simulink model "complete_plant_ediff_conflict_copy_Ethan’s MacBook Pro_2022_11_12"  (R2022b)
settings: Solver=FixedStepAuto  StartTime=0.0  StopTime=300  RelTol=1e-3  EnableMultiTasking=on
model workspace (MAT data in the model file):
  A = 1.0221
  A1 = Simulink.Parameter
  A1.Value = 39.8344
  A1.DataType = 'auto'
  A1.Complexity = 'real'
  A1.Dimensions = [1 1]
  A2 = Simulink.Parameter
  A2.Value = 813.078
  A2.DataType = 'auto'
  A2.Complexity = 'real'
  A2.Dimensions = [1 1]
  ALL_TRACK_DATA.track_data_Left = [Inf Inf Inf Inf Inf Inf Inf Inf Inf Inf Inf Inf ... (182152 elements, 22769x8)]
  ALL_TRACK_DATA.track_data_Right = [Inf Inf Inf Inf Inf Inf Inf Inf Inf Inf Inf Inf ... (182152 elements, 22769x8)]
  ALL_TRACK_DATA.track_data_acceleration = [Inf Inf Inf Inf Inf Inf Inf Inf Inf Inf Inf Inf ... (6008 elements, 751x8)]
  ALL_TRACK_DATA.track_data_endurance = [Inf -1348.33962917 -674.16944376 -449.445883811 -337.083980227 -269.666739189 -224.721829424 -192.618251815 -168.540506804 -149.813316856 -134.831515454 -122.573632994 ... (77796 elements, 19449x4)]
  ALL_TRACK_DATA.track_data_grand_prix = [Inf Inf Inf Inf Inf Inf Inf Inf Inf Inf Inf Inf ... (33752 elements, 4219x8)]
  ALL_TRACK_DATA.track_data_skidpad = [Inf Inf Inf Inf Inf Inf Inf Inf Inf Inf Inf Inf ... (18312 elements, 2289x8)]
  Af = 1.0221
  B1 = Simulink.Parameter
  B1.Value = 1.287e-06
  B1.DataType = 'auto'
  B1.Complexity = 'real'
  B1.Dimensions = [1 1]
  B2 = Simulink.Parameter
  B2.Value = -0.002325
  B2.DataType = 'auto'
  B2.Complexity = 'real'
  B2.Dimensions = [1 1]
  B3 = Simulink.Parameter
  B3.Value = 3.797
  B3.DataType = 'auto'
  B3.Complexity = 'real'
  B3.Dimensions = [1 1]
  BattCap = 16
  BattCap_I = 16
  C1 = Simulink.Parameter
  C1.Value = -2.541e-09
  C1.DataType = 'auto'
  C1.Complexity = 'real'
  C1.Dimensions = [1 1]
  C2 = Simulink.Parameter
  C2.Value = 5.279e-06
  C2.DataType = 'auto'
  C2.Complexity = 'real'
  C2.Dimensions = [1 1]
  C3 = Simulink.Parameter
  C3.Value = -0.003943
  C3.DataType = 'auto'
  C3.Complexity = 'real'
  C3.Dimensions = [1 1]
  C4 = Simulink.Parameter
  C4.Value = 3.634
  C4.DataType = 'auto'
  C4.Complexity = 'real'
  C4.Dimensions = [1 1]
  C_param = Simulink.Parameter
  C_param.Value = [0 13757.41 21278.97 26666.02 30253.47 30313.18 30313.18]
  C_param.DataType = 'auto'
  C_param.Complexity = 'real'
  C_param.Dimensions = [1 7]
  Cd = 1.149
  FZ_C = Simulink.Parameter
  FZ_C.Value = [0 204.13 427.04 668.1 895.72 1124.4 1324.4]
  FZ_C.DataType = 'auto'
  FZ_C.Complexity = 'real'
  FZ_C.Dimensions = [1 7]
  Fx_limit = Simulink.Parameter
  Fx_limit.Value = [300 300]
  Fx_limit.DataType = 'auto'
  Fx_limit.Complexity = 'real'
  Fx_limit.Dimensions = [1 2]
  I = Simulink.Parameter
  I.Value = 60
  I.DataType = 'auto'
  I.Complexity = 'real'
  I.Dimensions = [1 1]
  IYY_Tire = 0.3
  J_z = Simulink.Parameter
  J_z.Value = 75
  J_z.DataType = 'auto'
  J_z.Complexity = 'real'
  J_z.Dimensions = [1 1]
  Ku = Simulink.Parameter
  Ku.Value = 0.0509683995923
  Ku.DataType = 'auto'
  Ku.Complexity = 'real'
  Ku.Dimensions = [1 1]
  Motor_T_I = [30 30]
  Np = 4
  Ns = 80
  P = Simulink.Parameter
  P.Value = 3
  P.DataType = 'auto'
  P.Complexity = 'real'
  P.Dimensions = [1 1]
  RE = Simulink.Parameter
  RE.Value = 0.2228169203
  RE.DataType = 'auto'
  RE.Complexity = 'real'
  RE.Dimensions = [1 1]
  RIM_RADIUS = 0.1524
  Rm = 0.079375
  S1 = Simulink.Parameter
  S1.Value = 7e-05
  S1.DataType = 'auto'
  S1.Complexity = 'real'
  S1.Dimensions = [1 1]
  S2 = Simulink.Parameter
  S2.Value = -0.0038
  S2.DataType = 'auto'
  S2.Complexity = 'real'
  S2.Dimensions = [1 1]
  S3 = Simulink.Parameter
  S3.Value = 0.6535
  S3.DataType = 'auto'
  S3.Complexity = 'real'
  S3.Dimensions = [1 1]
  S4 = Simulink.Parameter
  S4.Value = 0.1061
  S4.DataType = 'auto'
  S4.Complexity = 'real'
  S4.Dimensions = [1 1]
  SL_limit = Simulink.Parameter
  SL_limit.Value = 0.3
  SL_limit.DataType = 'auto'
  SL_limit.Complexity = 'real'
  SL_limit.Dimensions = [1 1]
  T = Simulink.Parameter
  T.Value = 0
  T.DataType = 'single'
  T.Complexity = 'real'
  T.Dimensions = [1 1]
  T2F = Simulink.Parameter
  T2F.Value = [4.38500022888 4.38500022888 4.38500022888 4.38500022888]
  T2F.DataType = 'single'
  T2F.Complexity = 'real'
  T2F.Dimensions = [1 4]
  Tair = 293
  V_target = Simulink.Parameter
  V_target.Value = [0 3 6 9 12 15 18 21 25 31]
  V_target.DataType = 'auto'
  V_target.Complexity = 'real'
  V_target.Dimensions = [1 10]
  Vg_ref = 10
  Vth = Simulink.Parameter
  Vth.Value = 2
  Vth.DataType = 'auto'
  Vth.Complexity = 'real'
  Vth.Dimensions = [1 1]
  Vx_I = 0
  Vy_I = 0
  WHEEL_WIDTH = 0.1524
  a = Simulink.Parameter
  a.Value = 1.14
  a.DataType = 'auto'
  a.Complexity = 'real'
  a.Dimensions = [1 1]
  abs_max_torque = Simulink.Parameter
  abs_max_torque.Value = [25 25 25 25]
  abs_max_torque.DataType = 'auto'
  abs_max_torque.Complexity = 'real'
  abs_max_torque.Dimensions = [1 4]
  absolute_battery_power_limits = Simulink.Parameter
  absolute_battery_power_limits.Value = [75000 -700]
  absolute_battery_power_limits.DataType = 'auto'
  absolute_battery_power_limits.Complexity = 'real'
  absolute_battery_power_limits.Dimensions = [1 2]
  b = Simulink.Parameter
  b.Value = -0.03291
  b.DataType = 'auto'
  b.Complexity = 'real'
  b.Dimensions = [1 1]
  brake_bias = [0.65 0.65 0.35 0.35]
  brakecoeff = Simulink.Parameter
  brakecoeff.Value = [61.33 61.33 40.54 40.54]
  brakecoeff.DataType = 'auto'
  brakecoeff.Complexity = 'real'
  brakecoeff.Dimensions = [1 4]
  c = Simulink.Parameter
  c.Value = -1.14
  c.DataType = 'auto'
  c.Complexity = 'real'
  c.Dimensions = [1 1]
  cl = 2.11014
  d = Simulink.Parameter
  d.Value = -1.027
  d.DataType = 'auto'
  d.Complexity = 'real'
  d.Dimensions = [1 1]
  dTx = Simulink.Parameter
  dTx.Value = 0.01
  dTx.DataType = 'auto'
  dTx.Complexity = 'real'
  dTx.Dimensions = [1 1]
  dZ = 0.295
  d_bore = 0.0254
  deadband_angle = Simulink.Parameter
  deadband_angle.Value = 4
  deadband_angle.DataType = 'auto'
  deadband_angle.Complexity = 'real'
  deadband_angle.Dimensions = [1 1]
  deadband_velocity = Simulink.Parameter
  deadband_velocity.Value = 0.5
  deadband_velocity.DataType = 'auto'
  deadband_velocity.Complexity = 'real'
  deadband_velocity.Dimensions = [1 1]
  deg2rad = Simulink.Parameter
  deg2rad.Value = 0.01745329
  deg2rad.DataType = 'auto'
  deg2rad.Complexity = 'real'
  deg2rad.Dimensions = [1 1]
  di2bp = 20
  distance_traveled = 75
  efficiency_grid = Simulink.Parameter
  efficiency_grid.Value = [0.011 0.0107113163972 0.0104226327945 0.0101339491917 0.01 0.01 0.01 0.01 0.01 0.01 0.01 0.01 ... (26857 elements, 107x251)]
  efficiency_grid.DataType = 'auto'
  efficiency_grid.Complexity = 'real'
  efficiency_grid.Dimensions = [107 251]
  g = Simulink.Parameter
  g.Value = 9.81
  g.DataType = 'auto'
  g.Complexity = 'real'
  g.Dimensions = [1 1]
  gr = Simulink.Parameter
  gr.Value = [6.63043 6.63043 8 8]
  gr.DataType = 'auto'
  gr.Complexity = 'real'
  gr.Dimensions = [1 4]
  inch2mm = Simulink.Parameter
  inch2mm.Value = 25.4
  inch2mm.DataType = 'auto'
  inch2mm.Complexity = 'real'
  inch2mm.Dimensions = [1 1]
  k_limit = Simulink.Parameter
  k_limit.Value = 3.461
  k_limit.DataType = 'auto'
  k_limit.Complexity = 'real'
  k_limit.Dimensions = [1 1]
  kx = 200
  l = Simulink.Parameter
  l.Value = [0.7922471 0.7828529]
  l.DataType = 'auto'
  l.Complexity = 'real'
  l.Dimensions = [1 2]
  lateral_coeff = Simulink.Parameter
  lateral_coeff.Value = 1
  lateral_coeff.DataType = 'auto'
  lateral_coeff.Complexity = 'real'
  lateral_coeff.Dimensions = [1 1]
  m = 320
  m_tire_f = 6
  m_tire_r = 16
  max_delta_omega = Simulink.Parameter
  max_delta_omega.Value = 5
  max_delta_omega.DataType = 'auto'
  max_delta_omega.Complexity = 'real'
  max_delta_omega.Dimensions = [1 1]
  max_motor_temp = Simulink.Parameter
  max_motor_temp.Value = 75
  max_motor_temp.DataType = 'auto'
  max_motor_temp.Complexity = 'real'
  max_motor_temp.Dimensions = [1 1]
  max_rpm = Simulink.Parameter
  max_rpm.Value = [0 841.626809471 843.653762207 845.894764963 848.156711672 850.460546282 852.795796818 855.162463281 857.571017646 860.010987937 862.492846131 865.016592226 867.582226224 870.189748124 872.839157925 875.530455629 878.274113209 881.070130668 883.908036029 886.798301266 889.740926382 892.735911375 895.793728221 898.903904944 902.076913521 905.302281975 908.590482282 911.941514442 915.355378455 918.832074321 922.37160204 925.984433588 929.670568964 933.419536193 937.252279226 941.147854111 945.116732826 949.169387344 953.295345691 957.494607867 961.777645846 970.595049217 975.129414609 979.747555804 984.449472804 989.245637583 994.125578166 999.099766529 1004.16820267 1009.33088659 1014.58781829 1019.93899777 1025.39489701 1030.94504402 1036.58943882 1042.34902534 1048.20285965 1054.16141371 1060.2351595 1066.41362504 1072.69681034 1079.09518737 1085.59828416 1092.21657267 1098.95005292 1105.80919687 1112.77306058 1138.42940056]
  max_rpm.DataType = 'auto'
  max_rpm.Complexity = 'real'
  max_rpm.Dimensions = [1 68]
  max_torque = Simulink.Parameter
  max_torque.Value = [25 25 24.669 24.305 23.939 23.571 23.202 22.83 22.458 22.084 21.708 21.331 20.953 20.574 20.194 19.813 19.431 19.048 18.665 18.281 17.897 17.512 17.127 16.742 16.356 15.971 15.586 15.2 14.815 14.431 14.047 13.663 13.28 12.897 12.516 12.135 11.755 11.376 10.999 10.622 10.247 9.501 9.131 8.762 8.395 8.029 7.666 7.305 6.946 6.589 6.234 5.882 5.532 5.185 4.84 4.499 4.16 3.824 3.491 3.161 2.834 2.511 2.191 1.875 1.562 1.252 0.947 0]
  max_torque.DataType = 'auto'
  max_torque.Complexity = 'real'
  max_torque.Dimensions = [1 68]
  max_yaw_field = Simulink.Parameter
  max_yaw_field.Value = [0.67 0.67 0.67 0.83 0.57 0.62 0.377 0.4245 0.425 0.425]
  max_yaw_field.DataType = 'auto'
  max_yaw_field.Complexity = 'real'
  max_yaw_field.Dimensions = [1 10]
  mcp_Motor = 573
  min_velocity_regen = Simulink.Parameter
  min_velocity_regen.Value = 1.4
  min_velocity_regen.DataType = 'auto'
  min_velocity_regen.Complexity = 'real'
  min_velocity_regen.Dimensions = [1 1]
  motor_efficiency = Simulink.Parameter
  motor_efficiency.Value = [0.95 0.95 0.95 0.95]
  motor_efficiency.DataType = 'auto'
  motor_efficiency.Complexity = 'real'
  motor_efficiency.Dimensions = [1 4]
  motor_enable = Simulink.Parameter
  motor_enable.Value = [0 0 1 1]
  motor_enable.DataType = 'auto'
  motor_enable.Complexity = 'real'
  motor_enable.Dimensions = [1 4]
  mu_factor = Simulink.Parameter
  mu_factor.Value = 0.7
  mu_factor.DataType = 'auto'
  mu_factor.Complexity = 'real'
  mu_factor.Dimensions = [1 1]
  mu_k_brake = 0.4
  mu_s_brake = 0.5
  power_input_grid = Simulink.Parameter
  power_input_grid.Value = [0 0 0 0 0 0 0 0 0 0 0 0 ... (26857 elements, 251x107)]
  power_input_grid.DataType = 'auto'
  power_input_grid.Complexity = 'real'
  power_input_grid.Dimensions = [251 107]
  power_loss_grid = Simulink.Parameter
  power_loss_grid.Value = [0.1 0.2 0.3 0.4 0.5 0.6 0.7 0.8 0.9 1 1.1 1.2 ... (26857 elements, 251x107)]
  power_loss_grid.DataType = 'auto'
  power_loss_grid.Complexity = 'real'
  power_loss_grid.Dimensions = [251 107]
  power_loss_limit = Simulink.Parameter
  power_loss_limit.Value = [0 0 5800 5800]
  power_loss_limit.DataType = 'auto'
  power_loss_limit.Complexity = 'real'
  power_loss_limit.Dimensions = [1 4]
  rho = 1.225
  rpm_index_calibration = Simulink.Parameter
  rpm_index_calibration.Value = 10.4719755
  rpm_index_calibration.DataType = 'auto'
  rpm_index_calibration.Complexity = 'real'
  rpm_index_calibration.Dimensions = [1 1]
  rpm_sweep = Simulink.Parameter
  rpm_sweep.Value = [0 10.4719755 20.943951 31.4159265 41.887902 52.3598775 62.831853 73.3038285 83.775804 94.2477795 104.719755 115.1917305 125.663706 136.1356815 146.607657 157.0796325 167.551608 178.0235835 188.495559 198.9675345 209.43951 219.9114855 230.383461 240.8554365 251.327412 261.7993875 272.271363 282.7433385 293.215314 303.6872895 314.159265 324.6312405 335.103216 345.5751915 356.047167 366.5191425 376.991118 387.4630935 397.935069 408.4070445 418.87902 429.3509955 439.822971 450.2949465 460.766922 471.2388975 481.710873 492.1828485 502.654824 513.1267995 523.598775 534.0707505 544.542726 555.0147015 565.486677 575.9586525 586.430628 596.9026035 607.374579 617.8465545 628.31853 638.7905055 649.262481 659.7344565 670.206432 680.6784075 691.150383 701.6223585 712.094334 722.5663095 733.038285 743.5102605 753.982236 764.4542115 774.926187 785.3981625 795.870138 806.3421135 816.814089 827.2860645 837.75804 848.2300155 858.701991 869.1739665 879.645942 890.1179175 900.589893 911.0618685 921.533844 932.0058195 942.477795 952.9497705 963.421746 973.8937215 984.365697 994.8376725 1005.309648 1015.7816235 1026.253599 1036.7255745 1047.19755 1057.6695255 1068.141501 1078.6134765 1089.085452 1099.5574275 1110.029403]
  rpm_sweep.DataType = 'auto'
  rpm_sweep.Complexity = 'real'
  rpm_sweep.Dimensions = [1 107]
  s = Simulink.Parameter
  s.Value = [0.647895 0.62102]
  s.DataType = 'auto'
  s.Complexity = 'real'
  s.Dimensions = [1 2]
  steer_slope = Simulink.Parameter
  steer_slope.Value = 0.0111
  steer_slope.DataType = 'auto'
  steer_slope.Complexity = 'real'
  steer_slope.Dimensions = [1 1]
  t = Simulink.Parameter
  t.Value = 0.015
  t.DataType = 'auto'
  t.Complexity = 'real'
  t.Dimensions = [1 1]
  tau = Simulink.Parameter
  tau.Value = 0.0035
  tau.DataType = 'auto'
  tau.Complexity = 'real'
  tau.Dimensions = [1 1]
  time_delay = 0.022
  torque_sweep = Simulink.Parameter
  torque_sweep.Value = [0 0.1 0.2 0.3 0.4 0.5 0.6 0.7 0.8 0.9 1 1.1 1.2 1.3 1.4 1.5 1.6 1.7 1.8 1.9 2 2.1 2.2 2.3 2.4 2.5 2.6 2.7 2.8 2.9 3 3.1 3.2 3.3 3.4 3.5 3.6 3.7 3.8 3.9 4 4.1 4.2 4.3 4.4 4.5 4.6 4.7 4.8 4.9 5 5.1 5.2 5.3 5.4 5.5 5.6 5.7 5.8 5.9 6 6.1 6.2 6.3 6.4 6.5 6.6 6.7 6.8 6.9 7 7.1 7.2 7.3 7.4 7.5 7.6 7.7 7.8 7.9 8 8.1 8.2 8.3 8.4 8.5 8.6 8.7 8.8 8.9 9 9.1 9.2 9.3 9.4 9.5 9.6 9.7 9.8 9.9 10 10.1 10.2 10.3 10.4 10.5 10.6 10.7 10.8 10.9 11 11.1 11.2 11.3 11.4 11.5 11.6 11.7 11.8 11.9 12 12.1 12.2 12.3 12.4 12.5 12.6 12.7 12.8 12.9 13 13.1 13.2 13.3 13.4 13.5 13.6 13.7 13.8 13.9 14 14.1 14.2 14.3 14.4 14.5 14.6 14.7 14.8 14.9 15 15.1 15.2 15.3 15.4 15.5 15.6 15.7 15.8 15.9 16 16.1 16.2 16.3 16.4 16.5 16.6 16.7 16.8 16.9 17 17.1 17.2 17.3 17.4 17.5 17.6 17.7 17.8 17.9 18 18.1 18.2 18.3 18.4 18.5 18.6 18.7 18.8 18.9 19 19.1 19.2 19.3 19.4 19.5 19.6 19.7 19.8 19.9 20 20.1 20.2 20.3 20.4 20.5 20.6 20.7 20.8 20.9 21 21.1 21.2 21.3 21.4 21.5 21.6 21.7 21.8 21.9 22 22.1 22.2 22.3 22.4 22.5 22.6 22.7 22.8 22.9 23 23.1 23.2 23.3 23.4 23.5 23.6 23.7 23.8 23.9 24 24.1 24.2 24.3 24.4 24.5 24.6 24.7 24.8 24.9 25]
  torque_sweep.DataType = 'auto'
  torque_sweep.Complexity = 'real'
  torque_sweep.Dimensions = [1 251]
  track_type = 1
  voltage_grid = Simulink.Parameter
  voltage_grid.Value = [0 0 0 0 0 0 0 0 0 0 0 0 ... (26857 elements, 251x107)]
  voltage_grid.DataType = 'auto'
  voltage_grid.Complexity = 'real'
  voltage_grid.Dimensions = [251 107]
  yaw_I = 0
  yaw_deadband = Simulink.Parameter
  yaw_deadband.Value = 1
  yaw_deadband.DataType = 'auto'
  yaw_deadband.Complexity = 'real'
  yaw_deadband.Dimensions = [1 1]
  yaw_error_limit = Simulink.Parameter
  yaw_error_limit.Value = 0.2
  yaw_error_limit.DataType = 'auto'
  yaw_error_limit.Complexity = 'real'
  yaw_error_limit.Dimensions = [1 1]
undefined symbols (not defined in the file): accel, ang, ang_vel, battery_voltage, brake_pressure, DiscIntNeverNeededParam, Driver, driver_input, F0z, FZ, motor_T, omega, power_limits, Reference, shock_displacement, shock_velocity, steering_angle, VEH, vel
libraries: fl_lib x20, nesl_utility x12, vehdynlibtire x10, vehdynlibsuspension x8, autolibutils x5, sharedtransform x5, sdl_lib x4, slpidlib x2, shared6dof x2, simulink x1, autolibdatasheetbattery x1, autolibmappedmotor x1
(part 1 of 10)
settings Model: Creator=Inver  LastModifiedBy=ethanharris
settings SolverCC: AutoInsertRateTranBlk=on
settings DataIOCC: ReturnWorkspaceOutputsName=tpb23fdb8c_83dd_4bc7_9121_68f18caf90f2
settings OptimizationCC: DefaultParameterBehavior=Inlined  UseDivisionForNetSlopeComputation=on  GainParamInheritBuiltInType=on  UseFloatMulNetSlope=on  UseSpecifiedMinMax=on  InlineInvariantSignals=on  StrengthReduction=on  ZeroExternalMemoryAtStartup=off  ZeroInternalMemoryAtStartup=off  NoFixptDivByZeroProtection=on  EfficientFloat2IntCast=on  LifeSpan=1  MaxStackSize=64  OptimizeBlockOrder=speed  OptimizationPriority=Speed  OptimizationCustomize=off  MultiThreadedLoops=on  EfficientTunableParamExpr=on
settings DebuggingCC: ParameterTunabilityLossMsg=error
settings HardwareCC: ProdBitPerPointer=32  ProdBitPerSizeT=32  ProdBitPerPtrDiffT=32  ProdLargestAtomicInteger=Long  ProdLargestAtomicFloat=Double  ProdWordSize=32  ProdLongLongMode=on  ProdHWDeviceType=ARM Compatible->ARM Cortex-M
settings ModelReferenceCC: EnableRefExpFcnMdlSchedulingChecks=on
settings SFSimCC: SimCustomHeaderCode="#include \"eDiff.h\""  SimUserSources=eDiff.c  MATLABDynamicMemAlloc=off
settings RTWCC: Description=Embedded Coder  SystemTargetFile=ert.tlc  GenCodeOnly=on  PackageGeneratedCodeAndArtifacts=on  PackageName=TVS_CODE  TemplateMakefile=ert_default_tmf  Toolchain=GNU Tools for ARM Embedded Processors  BuildConfiguration=Faster Runs  CodeExecutionProfiling=on  CodeProfilingInstrumentation=detailed
settings CodeAppCC: ForceParamTrailComments=on  IgnoreCustomStorageClasses=off  OperatorAnnotations=on  SimulinkDataObjDesc=on  SFDataObjDesc=on  CustomSymbolStrGlobalVar=rt$N$M  CustomSymbolStrType=$N$M  CustomSymbolStrFcn=$N$M$F  CustomSymbolStrMacro=$N$M  InsertBlockDesc=on
settings ERTTargetCC: GenerateSampleERTMain=on  IncludeMdlTerminateFcn=off  CombineSignalStateStructs=on  CodeInterfacePackaging=Reusable function  SupportNonFinite=off  SupportComplex=off  SupportNonInlinedSFcns=on  InlinedParameterPlacement=NonHierarchical  RootIOFormat=Structure reference  ERTCustomFileTemplate=example_file_process.tlc  GlobalDataDefinition=InSeparateSourceFile  DataDefinitionFile=data.c  GlobalDataReference=InSeparateHeaderFile  ERTFilePackagingFormat=CompactWithDataFile  DataReferenceFile=data.h

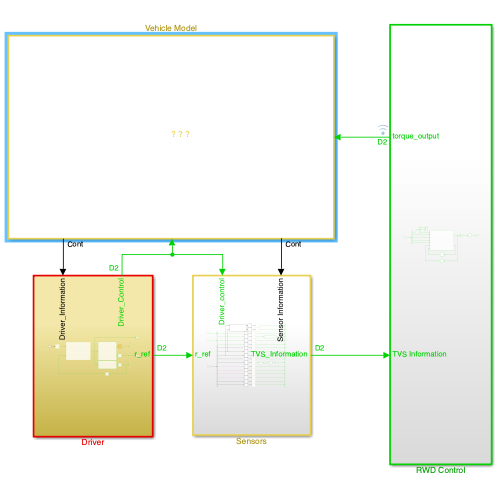
[thumbnail: Simulink's stored preview of the top-level diagram]
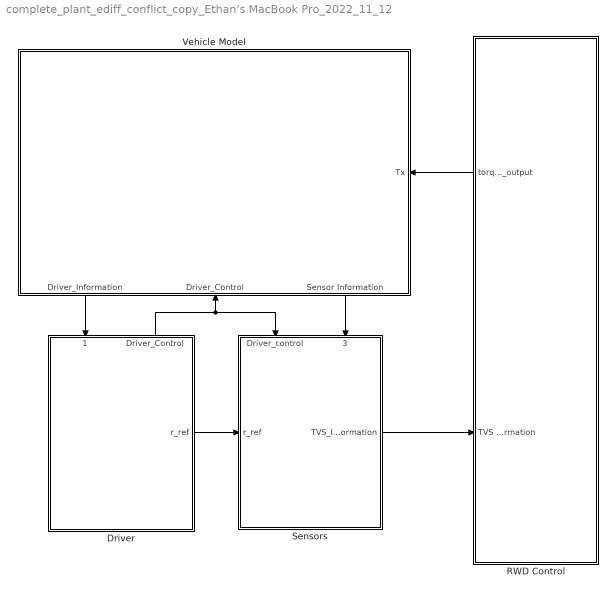
== system complete_plant_ediff_conflict_copy_Ethan’s MacBook Pro_2022_11_12 ==
  Driver : Subsystem  TreatAsAtomicUnit=on
      settings: PortSchema="{\"entries\":[{\"content\":{\"sides\":[{\"content\":{\"connectorIds\":[]},\"type\":\"ConnectorPlacement.EquallySpacedRectSide\",\"uuid\":\"bd499254-800d-4f65-9d66-206e4f6126a9\"},{\"content\":{\"connectorIds\":[\"Out1\"],\"side\":\"RIGHT\"},\"type\":\"ConnectorPlacement.EquallySpacedRectSide\",\"uuid\":\"787bb70a-048d-46a8-9404-9c629bdce5fb\"},{\"content\":{\"connectorIds\":[\"In1\",\"Out2\"],\"side\":\"TOP\"},\"type\":\"ConnectorPlacement.EquallySpacedRectSide\",\"uuid\":\"94a1f635-0878-46b0-949b-f2a3fa746134\"}]},\"type\":\"ConnectorPlacement.EquallySpacedConnector\",\"uuid\":\"f81a85a8-63b1-46ab-bae2-7f37115d6b57\"}],\"packageUris\":[\"http://schema.mathworks.com/mf0/Connector/R2020b\"],\"version\":\"1.0\"}"
  RWD Control : Subsystem  TreatAsAtomicUnit=on
      settings: PortSchema="{\"entries\":[{\"content\":{\"sides\":[{\"content\":{\"connectorIds\":[\"Out1\",\"In1\"]},\"type\":\"ConnectorPlacement.EquallySpacedRectSide\",\"uuid\":\"055d7d7f-e9cc-48e9-8f01-9f88989d1e3a\"},{\"content\":{\"connectorIds\":[],\"side\":\"RIGHT\"},\"type\":\"ConnectorPlacement.EquallySpacedRectSide\",\"uuid\":\"cd4df1f5-4977-418c-b4c3-79190dfdd2e9\"},{\"content\":{\"connectorIds\":[],\"side\":\"TOP\"},\"type\":\"ConnectorPlacement.EquallySpacedRectSide\",\"uuid\":\"259ba1a5-5484-4a84-a4e5-668874c69fd0\"},{\"content\":{\"connectorIds\":[],\"side\":\"BOTTOM\"},\"type\":\"ConnectorPlacement.EquallySpacedRectSide\",\"uuid\":\"06ba949a-0766-4c39-aac4-4f388039a879\"},{\"content\":{\"connectorIds\":[],\"side\":\"HIDDEN\"},\"type\":\"ConnectorPlacement.EquallySpacedRectSide\",\"uuid\":\"3b3d1b4f-8e5f-479c-975d-a63ab17a3080\"}]},\"type\":\"ConnectorPlacement.EquallySpacedConnector\",\"uuid\":\"a90ae5ed-4113-4a01-be54-d21f6ba2c1d4\"}],\"packageUris\":[\"http://schema.mathworks.com/mf0/Connector/R2020b\"],\"version\":\"1.0\"}"
  Sensors : Subsystem  TreatAsAtomicUnit=on
      settings: PortSchema="{\"entries\":[{\"content\":{\"sides\":[{\"content\":{\"connectorIds\":[\"In1\"]},\"type\":\"ConnectorPlacement.EquallySpacedRectSide\",\"uuid\":\"bd499254-800d-4f65-9d66-206e4f6126a9\"},{\"content\":{\"connectorIds\":[\"Out1\"],\"side\":\"RIGHT\"},\"type\":\"ConnectorPlacement.EquallySpacedRectSide\",\"uuid\":\"787bb70a-048d-46a8-9404-9c629bdce5fb\"},{\"content\":{\"connectorIds\":[\"In2\",\"In3\"],\"side\":\"TOP\"},\"type\":\"ConnectorPlacement.EquallySpacedRectSide\",\"uuid\":\"94a1f635-0878-46b0-949b-f2a3fa746134\"}]},\"type\":\"ConnectorPlacement.EquallySpacedConnector\",\"uuid\":\"f81a85a8-63b1-46ab-bae2-7f37115d6b57\"}],\"packageUris\":[\"http://schema.mathworks.com/mf0/Connector/R2020b\"],\"version\":\"1.0\"}"
  Vehicle Model : Subsystem  TreatAsAtomicUnit=on
      settings: PortSchema="{\"entries\":[{\"content\":{\"sides\":[{\"content\":{\"connectorIds\":[]},\"type\":\"ConnectorPlacement.EquallySpacedRectSide\",\"uuid\":\"7263df3d-11c2-488e-998f-6bd776306b9c\"},{\"content\":{\"connectorIds\":[\"In2\"],\"side\":\"RIGHT\"},\"type\":\"ConnectorPlacement.EquallySpacedRectSide\",\"uuid\":\"b0de89c2-35d2-4c59-81fc-f1f509ccf522\"},{\"content\":{\"connectorIds\":[],\"side\":\"TOP\"},\"type\":\"ConnectorPlacement.EquallySpacedRectSide\",\"uuid\":\"474ba072-8402-41d1-8015-97ca573757b9\"},{\"content\":{\"connectorIds\":[\"Out1\",\"In1\",\"Out2\"],\"side\":\"BOTTOM\"},\"type\":\"ConnectorPlacement.EquallySpacedRectSide\",\"uuid\":\"2efad9e8-b0d8-4de5-bddc-0b63eaa22f81\"}]},\"type\":\"ConnectorPlacement.EquallySpacedConnector\",\"uuid\":\"426f55ca-7f3f-41f0-94e6-91e6d6304a5e\"}],\"packageUris\":[\"http://schema.mathworks.com/mf0/Connector/R2020b\"],\"version\":\"1.0\"}"
      mask Display: image('C:\Users\Inver\MATLAB Drive\Top Model - Master\Bling\PER22.png'); % Use "Edit Image" on toolstrip to change.
  wires:
  Vehicle Model/1(Driver_Information) -> Driver/1(Driver_Information)
  Vehicle Model/2(Sensor Information) -> Sensors/3(Sensor Information)
  Driver/2(Driver_Control) -> Vehicle Model/1(Driver_Control), Sensors/2(Driver_control)
  Sensors/1(TVS_Information) -> RWD Control/1(TVS Information)
  RWD Control/1(torque_output) -> Vehicle Model/2(Tx)
  Driver/1(r_ref) -> Sensors/1(r_ref)

== system complete_plant_ediff_conflict_copy_Ethan’s MacBook Pro_2022_11_12/Driver ==
  Driver_Information : Inport
  Bus Creator : BusCreator  Inputs=driver_input,brake_pressure,steering_angle
  Lateral Control : Subsystem
  Longitudinal Control : Subsystem
  Rate Transition : RateTransition  OutPortSampleTime=t
  Reference Generator : Subsystem
  Unit Delay{,1..3} (4 alike) : UnitDelay  SampleTime=-1  HasFrameUpgradeWarning=on
  r_ref : Outport  SampleTime=t
  Driver_Control : Outport  Port=2  SampleTime=t
  wires:
  Longitudinal Control/1(driver_input) -> Unit Delay3/1
  Bus Creator/1 -> Driver_Control/1
  Longitudinal Control/2(brake_pressure) -> Unit Delay2/1
  Reference Generator/1(Controller Information) -> r_ref/1, Lateral Control/1(Controller Information), Longitudinal Control/1(Controller Information)
  Rate Transition/1 -> Reference Generator/1(Driver_Information)  "driver_input"
  Driver_Information/1 -> Rate Transition/1
  Lateral Control/1(steering_angle) -> Unit Delay1/1
  Unit Delay/1 -> Reference Generator/2(steering_angle)
  Unit Delay2/1 -> Bus Creator/2  "brake_pressure"
  Unit Delay1/1 -> Unit Delay/1, Bus Creator/3  "steering_angle"
  Unit Delay3/1 -> Bus Creator/1  "driver_input"

== system complete_plant_ediff_conflict_copy_Ethan’s MacBook Pro_2022_11_12/RWD Control ==
  TVS Information : Inport
  Bus Selector : BusSelector  OutputSignals=ang_vel,left_wheel_speed,right_wheel_speed,driver_input,steering_angle
  Demux4 : Demux  Outputs=3
  Gain : Gain  Gain=25/4095
  MATLAB Function : MATLAB Function  TreatAsAtomicUnit=on
  Rate Limiter : RateLimiter  RisingSlewLimit=125  FallingSlewLimit=-300  SampleTimeMode=inherited
  Terminator5 : Terminator
  Terminator6 : Terminator
  Unit Delay1 : UnitDelay  InitialCondition=[0 0 0 0]  SampleTime=-1  HasFrameUpgradeWarning=on
  Unit Delay3 : UnitDelay  SampleTime=-1  HasFrameUpgradeWarning=on
  torque_output : Outport
  wires:
  Bus Selector/4 -> MATLAB Function/4(AP)  "<driver_input>"
  Demux4/3 -> MATLAB Function/1(yaw)
  Bus Selector/5 -> MATLAB Function/5(sensor_steering_wheel_angle)  "<steering_angle>"
  Bus Selector/2 -> MATLAB Function/2(left_wheel_speed)  "<left_wheel_speed>"
  Bus Selector/3 -> MATLAB Function/3(right_wheel_speed)  "<right_wheel_speed>"
  MATLAB Function/1(Tx) -> Unit Delay1/1, Gain/1
  Unit Delay1/1 -> MATLAB Function/6(prev_Tx)
  Unit Delay3/1 -> MATLAB Function/7("filter_yaw ")
  MATLAB Function/2(filter_yaw) -> Unit Delay3/1
  Demux4/2 -> Terminator5/1
  Bus Selector/1 -> Demux4/1  "<ang_vel>"
  Demux4/1 -> Terminator6/1
  TVS Information/1 -> Bus Selector/1
  Gain/1 -> Rate Limiter/1
  Rate Limiter/1 -> torque_output/1

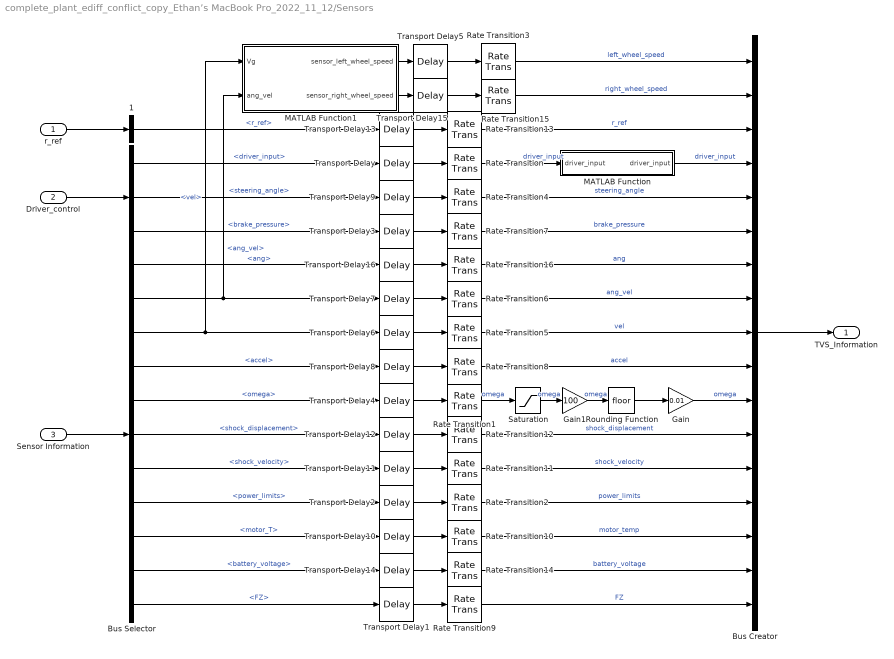
== system complete_plant_ediff_conflict_copy_Ethan’s MacBook Pro_2022_11_12/Sensors ==
  r_ref : Inport
  Driver_control : Inport  Port=2
  Sensor Information : Inport  Port=3
  " " : BusSelector  OutputSignals=driver_input,steering_angle,brake_pressure
  " 1" : BusSelector  OutputSignals=Reference.r_ref
  Bus Creator : BusCreator  Inputs=17
  Bus Selector : BusSelector  OutputSignals=ang,ang_vel,vel,accel,omega,shock_displacement,shock_velocity,power_limits,motor_T,battery_voltage,FZ
  Gain : Gain  Gain=0.01
  Gain1 : Gain  Gain=100
  MATLAB Function : MATLAB Function  TreatAsAtomicUnit=on
  MATLAB Function1 : MATLAB Function  TreatAsAtomicUnit=on
  Rate Transition{,3..4,13..15} (6 alike) : RateTransition  OutPortSampleTime=t
  Rate Transition{1,7,9..12} (6 alike) : RateTransition  InitialCondition=[0 0 0 0]  OutPortSampleTime=t
  Rate Transition16 : RateTransition  InitialCondition=[0 0 0]  OutPortSampleTime=t
  Rate Transition2 : RateTransition  InitialCondition=[0 0]  OutPortSampleTime=t
  Rate Transition5 : RateTransition  InitialCondition=[0 0]  OutPortSampleTime=t
  Rate Transition6 : RateTransition  InitialCondition=[0 0 0]  OutPortSampleTime=t
  Rate Transition8 : RateTransition  InitialCondition=[0 0 0]  OutPortSampleTime=t
  Rounding Function : Rounding
  Saturation : Saturate  UpperLimit=inf  LowerLimit=0
  Transport Delay{,5,9,13,15} (5 alike) : TransportDelay  DelayTime=time_delay  BufferSize=25000
  Transport Delay1 : TransportDelay  DelayTime=time_delay  InitialOutput=[750 750 750 750]  BufferSize=25000
  Transport Delay{3..4,10..12} (5 alike) : TransportDelay  DelayTime=time_delay  InitialOutput=[0 0 0 0]  BufferSize=25000
  Transport Delay14 : TransportDelay  DelayTime=time_delay  InitialOutput=336  BufferSize=25000
  Transport Delay16 : TransportDelay  DelayTime=time_delay  InitialOutput=[0 0 0]  BufferSize=25000
  Transport Delay2 : TransportDelay  DelayTime=time_delay  InitialOutput=[0 0]  BufferSize=25000
  Transport Delay6 : TransportDelay  DelayTime=time_delay  InitialOutput=[0 0]  BufferSize=25000
  Transport Delay7 : TransportDelay  DelayTime=time_delay  InitialOutput=[0 0 0]  BufferSize=25000
  Transport Delay8 : TransportDelay  DelayTime=time_delay  InitialOutput=[0 0 0]  BufferSize=25000
  TVS_Information : Outport
  wires:
  Transport Delay2/1 -> Rate Transition2/1
  Rate Transition8/1 -> Bus Creator/10  "accel"
  Transport Delay4/1 -> Rate Transition1/1
  Rate Transition12/1 -> Bus Creator/12  "shock_displacement"
  Rate Transition9/1 -> Bus Creator/17  "FZ"
  Bus Selector/2 -> Transport Delay7/1, MATLAB Function1/2(ang_vel)  "<ang_vel>"
  Bus Selector/5 -> Transport Delay4/1  "<omega>"
  Rate Transition11/1 -> Bus Creator/13  "shock_velocity"
  Rate Transition4/1 -> Bus Creator/5  "steering_angle"
  Transport Delay12/1 -> Rate Transition12/1
  Bus Selector/11 -> Transport Delay1/1  "<FZ>"
  Transport Delay9/1 -> Rate Transition4/1
  Transport Delay8/1 -> Rate Transition8/1
  Transport Delay1/1 -> Rate Transition9/1
  Bus Selector/7 -> Transport Delay11/1  "<shock_velocity>"
  Transport Delay11/1 -> Rate Transition11/1
  Transport Delay7/1 -> Rate Transition6/1
  " "/2 -> Transport Delay9/1  "<steering_angle>"
  Bus Selector/6 -> Transport Delay12/1  "<shock_displacement>"
  Rate Transition2/1 -> Bus Creator/14  "power_limits"
  Sensor Information/1 -> Bus Selector/1
  Transport Delay6/1 -> Rate Transition5/1
  Driver_control/1 -> " "/1
  Bus Selector/3 -> MATLAB Function1/1(Vg), Transport Delay6/1  "<vel>"
  Rate Transition5/1 -> Bus Creator/9  "vel"
  Rate Transition6/1 -> Bus Creator/8  "ang_vel"
  " "/1 -> Transport Delay/1  "<driver_input>"
  Transport Delay/1 -> Rate Transition/1
  Transport Delay3/1 -> Rate Transition7/1
  Rate Transition7/1 -> Bus Creator/6  "brake_pressure"
  " "/3 -> Transport Delay3/1  "<brake_pressure>"
  Bus Selector/8 -> Transport Delay2/1  "<power_limits>"
  Bus Creator/1 -> TVS_Information/1
  Rate Transition10/1 -> Bus Creator/15  "motor_temp"
  Transport Delay10/1 -> Rate Transition10/1
  Bus Selector/9 -> Transport Delay10/1  "<motor_T>"
  Gain/1 -> Bus Creator/11  "omega"
  Rate Transition1/1 -> Saturation/1  "omega"
  Rate Transition/1 -> MATLAB Function/1("driver_input ")  "driver_input"
  MATLAB Function/1(driver_input) -> Bus Creator/4  "driver_input"
  Saturation/1 -> Gain1/1  "omega"
  Rounding Function/1 -> Gain/1
  Gain1/1 -> Rounding Function/1  "omega"
  Transport Delay13/1 -> Rate Transition13/1
  Rate Transition13/1 -> Bus Creator/3  "r_ref"
  r_ref/1 -> " 1"/1
  " 1"/1 -> Transport Delay13/1  "<r_ref>"
  Transport Delay14/1 -> Rate Transition14/1
  Bus Selector/10 -> Transport Delay14/1  "<battery_voltage>"
  Rate Transition14/1 -> Bus Creator/16  "battery_voltage"
  Bus Selector/4 -> Transport Delay8/1  "<accel>"
  Transport Delay16/1 -> Rate Transition16/1
  Bus Selector/1 -> Transport Delay16/1  "<ang>"
  Rate Transition16/1 -> Bus Creator/7  "ang"
  Rate Transition15/1 -> Bus Creator/2  "right_wheel_speed"
  Rate Transition3/1 -> Bus Creator/1  "left_wheel_speed"
  Transport Delay5/1 -> Rate Transition3/1
  MATLAB Function1/1(sensor_left_wheel_speed) -> Transport Delay5/1
  Transport Delay15/1 -> Rate Transition15/1
  MATLAB Function1/2(sensor_right_wheel_speed) -> Transport Delay15/1

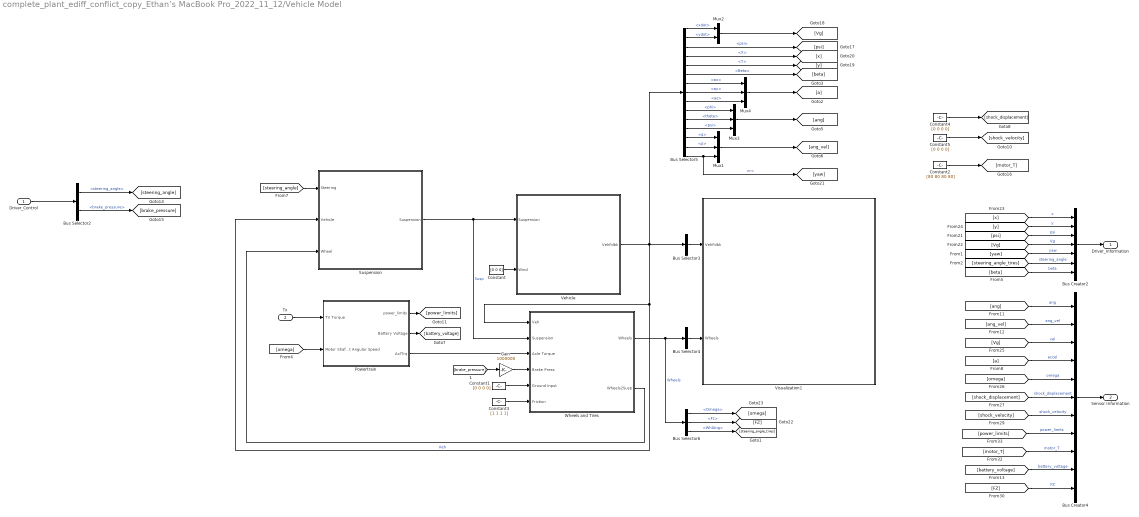
== system complete_plant_ediff_conflict_copy_Ethan’s MacBook Pro_2022_11_12/Vehicle Model ==
  Driver_Control : Inport
  Tx : Inport  Port=2
  Bus Creator2 : BusCreator  Inputs=7
  Bus Creator4 : BusCreator  Inputs=ang,ang_vel,vel,accel,omega,shock_displacement,shock_velocity,power_limits,motor_T,battery_voltage,FZ
  Bus Selector2 : BusSelector  OutputSignals=steering_angle,brake_pressure
  Bus Selector3 : BusSelector  OutputSignals=InertFrm,BdyFrm  OutputAsBus=on
  Bus Selector4 : BusSelector  OutputSignals=TireFrame,Steering  OutputAsBus=on
  Bus Selector5 : BusSelector  OutputSignals=BdyFrm.Cg.Vel.xdot,BdyFrm.Cg.Vel.ydot,InertFrm.Cg.Ang.psi,InertFrm.Cg.Disp.X,InertFrm.Cg.Disp.Y,BdyFrm.Cg.Ang.Beta,BdyFrm.Cg.Acc.ax,BdyFrm.Cg.Acc.ay,BdyFrm.Cg.Acc.az,InertFrm.Cg.Ang.phi,InertFrm.Cg.Ang.theta,InertFrm.Cg.Ang.psi,BdyFrm.Cg.AngVel.q,BdyFrm.Cg.AngVel.p,BdyFrm.Cg.AngVel.r
  Bus Selector6 : BusSelector  OutputSignals=TireFrame.Omega,TireFrame.Fz,Steering.WhlAng
  Constant : Constant  Value=[0 0 0]
  Constant1 : Constant  Value=[0 0 0 0]
  Constant2 : Constant  Value=[80 80 80 80]
  Constant3 : Constant  Value=[1 1 1 1]
  Constant4 : Constant  Value=[0 0 0 0]
  Constant5 : Constant  Value=[0 0 0 0]
  Gain : Gain  Gain=1000000
  Mux1 : Mux  Inputs=3
  Mux2 : Mux  Inputs=2
  Mux3 : Mux  Inputs=3
  Mux4 : Mux  Inputs=3
  Powertrain : Subsystem
  Suspension : Subsystem  Variant=on  VariantControlMode=label  LabelModeActiveChoice=1
      mask Display:
      | switch str2num(get_param(gcb,'ActiveVariant'))
      |     case 1
      |         image('suspdw.png');
      |     case 2
      |         image([imread('suspindmap.png');imread('suspsamap.png')]);
      |     case 3
      |          image([imread('suspmacp.png');imread('suspsacoil.png')]);
      |     case 4
      |          image('suspmacp.png');
      |     case 5
      |          image('suspindmap.png');
      |     case 6
      |          image('suspkandc.png');
      | end
  Vehicle : Subsystem
      mask Display: image('6dofcar.png');
  Visualization1 : Subsystem
  Wheels and Tires : Subsystem
      mask Display: image('wheel3dof.png')
  Driver_Information : Outport
  Sensor Information : Outport  Port=2
  wires:
  Constant5/1 -> [shock_velocity]
  Constant4/1 -> [shock_displacement]
  Driver_Control/1 -> Bus Selector2/1
  Bus Selector2/1 -> [steering_angle]  "<steering_angle>"
  Bus Selector2/2 -> [brake_pressure]  "<brake_pressure>"
  Constant2/1 -> [motor_T]
  Constant3/1 -> Wheels and Tires/6(Friction)
  Constant1/1 -> Wheels and Tires/5(Ground Input)
  Bus Selector3/1 -> Visualization1/1(VehFdbk)
  Suspension/1(Suspension) -> Vehicle/1(Suspension), Wheels and Tires/2(Suspension)  "Susp"
  Constant/1 -> Vehicle/2(Wind)
  Wheels and Tires/1(Wheels) -> Bus Selector6/1, Bus Selector4/1  "Wheels"
  Vehicle/1(VehFdbk) -> Bus Selector5/1, Bus Selector3/1, Wheels and Tires/1(Veh), Suspension/2(Vehicle)  "Veh"
  [steering_angle] -> Suspension/1(Steering)
  Wheels and Tires/2(Wheels2Susp) -> Suspension/3(Wheel)
  Bus Selector4/1 -> Visualization1/2(Wheels)
  Bus Selector5/15 -> Mux1/3, [yaw]  "<r>"
  Bus Selector5/3 -> [psi]  "<psi>"
  Bus Selector5/4 -> [x]  "<X>"
  Bus Selector5/5 -> [y]  "<Y>"
  Bus Selector6/1 -> [omega]  "<Omega>"
  Bus Selector6/2 -> [FZ]  "<Fz>"
  [x] -> Bus Creator2/1  "x"
  Bus Creator2/1 -> Driver_Information/1
  [psi] -> Bus Creator2/3  "psi"
  [Vg] -> Bus Creator2/4  "Vg"
  [y] -> Bus Creator2/2  "y"
  Bus Selector5/1 -> Mux2/1  "<xdot>"
  Mux2/1 -> [Vg]
  Bus Selector5/2 -> Mux2/2  "<ydot>"
  [shock_velocity] -> Bus Creator4/7  "shock_velocity"
  Bus Creator4/1 -> Sensor Information/1
  [shock_displacement] -> Bus Creator4/6  "shock_displacement"
  [ang_vel] -> Bus Creator4/2  "ang_vel"
  [motor_T] -> Bus Creator4/9  "motor_T"
  [power_limits] -> Bus Creator4/8  "power_limits"
  [Vg] -> Bus Creator4/3  "vel"
  Tx/1 -> Powertrain/1(TV Torque)
  [omega] -> Powertrain/2(Motor Shaft Angular Speed)
  Powertrain/1(power_limits) -> [power_limits]
  Powertrain/3(AxlTrq) -> Wheels and Tires/3(Axle Torque)
  [yaw] -> Bus Creator2/5  "yaw"
  Bus Selector6/3 -> [steering_angle_tires]  "<WhlAng>"
  [steering_angle_tires] -> Bus Creator2/6  "steering_angle"
  Gain/1 -> Wheels and Tires/4(Brake Press)
  [brake_pressure] -> Gain/1
  Bus Selector5/6 -> [beta]  "<Beta>"
  [beta] -> Bus Creator2/7  "beta"
  Bus Selector5/10 -> Mux3/1  "<phi>"
  Bus Selector5/11 -> Mux3/2  "<theta>"
  Bus Selector5/12 -> Mux3/3  "<psi>"
  Mux3/1 -> [ang]
  Bus Selector5/13 -> Mux1/1  "<q>"
  Bus Selector5/14 -> Mux1/2  "<p>"
  Mux1/1 -> [ang_vel]
  Powertrain/2(Battery Voltage) -> [battery_voltage]
  Bus Selector5/9 -> Mux4/3  "<az>"
  Bus Selector5/8 -> Mux4/2  "<ay>"
  Bus Selector5/7 -> Mux4/1  "<ax>"
  Mux4/1 -> [a]
  [ang] -> Bus Creator4/1  "ang"
  [a] -> Bus Creator4/4  "accel"
  [omega] -> Bus Creator4/5  "omega"
  [battery_voltage] -> Bus Creator4/10  "battery_voltage"
  [FZ] -> Bus Creator4/11  "FZ"

== system complete_plant_ediff_conflict_copy_Ethan’s MacBook Pro_2022_11_12/Driver/Lateral Control ==
  Controller Information : Inport
  Bus Selector : BusSelector  OutputSignals=Reference.r_error_2,Reference.d_error,Reference.v_cog,Reference.psi_error,Reference.wind_down
  Lateral Controller : Subsystem
  steering_angle : Outport
  wires:
  Controller Information/1 -> Bus Selector/1
  Bus Selector/2 -> Lateral Controller/2(d_error)  "<d_error>"
  Bus Selector/3 -> Lateral Controller/3(<Vg>)  "<v_cog>"
  Bus Selector/4 -> Lateral Controller/4(angle_error)  "<psi_error>"
  Lateral Controller/1(steering_angle) -> steering_angle/1
  Bus Selector/1 -> Lateral Controller/1(r_error)  "<r_error_2>"
  Bus Selector/5 -> Lateral Controller/5(wind_down)  "<wind_down>"

== system complete_plant_ediff_conflict_copy_Ethan’s MacBook Pro_2022_11_12/Driver/Longitudinal Control ==
  Controller Information : Inport
  Abs : Abs  SaturateOnIntegerOverflow=off
  Bus Selector : BusSelector  OutputSignals=Reference.v_error
  Constant : Constant
  Constant1 : Constant  Value=0.6
  Constant2 : Constant  Value=25
  Constant3 : Constant  Value=-5
  Constant4 : Constant  Value=-0.75
  Discrete-Time Integrator : DiscreteIntegrator  ExternalReset=rising  SampleTime=-1  LimitOutput=on  UpperSaturationLimit=1  LowerSaturationLimit=-1  ICPrevOutput=DiscIntNeverNeededParam  ICPrevScaledInput=DiscIntNeverNeededParam
  Gain : Gain  Gain=0.7
  Gain1 : Gain
  Less Than : RelationalOperator  Operator=<  OutDataTypeStr=boolean  RndMeth=Simplest  InputSameDT=off
  Less Than1 : RelationalOperator  Operator=<  OutDataTypeStr=boolean  RndMeth=Simplest  InputSameDT=off
  MATLAB Function : MATLAB Function  TreatAsAtomicUnit=on
  NOT : Logic  Operator=NOT  IconShape=distinctive  AllPortsSameDT=off  OutDataTypeStr=boolean
  Product : Product
  Rate Limiter : RateLimiter  RisingSlewLimit=100  SampleTimeMode=inherited
  Rate Limiter Dynamic : simulink/Discontinuities/Rate Limiter Dynamic
  Saturation : Saturate  UpperLimit=1  LowerLimit=-1
  Sum2 : Sum  Inputs=|++
  Switch : Switch  Criteria=u2 > Threshold  SaturateOnIntegerOverflow=off  InputSameDT=off
  driver_input : Outport  PortDimensions=1
  brake_pressure : Outport  Port=2
  wires:
  Gain1/1 -> Discrete-Time Integrator/1
  Gain/1 -> Sum2/1
  Product/1 -> Gain1/1
  Sum2/1 -> Saturation/1
  Constant/1 -> Less Than/2
  MATLAB Function/1(brake_pressure) -> brake_pressure/1
  Bus Selector/1 -> Product/1, Gain/1, Abs/1  "<v_error>"
  Abs/1 -> Less Than/1
  Less Than/1 -> NOT/1, Product/2
  NOT/1 -> Discrete-Time Integrator/2
  Saturation/1 -> Rate Limiter/1, Rate Limiter Dynamic/2
  Constant2/1 -> Rate Limiter Dynamic/1
  Rate Limiter Dynamic/1 -> MATLAB Function/1(driver_input), driver_input/1
  Less Than1/1 -> Switch/2
  Constant1/1 -> Less Than1/2
  Switch/1 -> Rate Limiter Dynamic/3
  Constant3/1 -> Switch/3
  Constant4/1 -> Switch/1
  Rate Limiter/1 -> Less Than1/1
  Controller Information/1 -> Bus Selector/1
  Discrete-Time Integrator/1 -> Sum2/2

== system complete_plant_ediff_conflict_copy_Ethan’s MacBook Pro_2022_11_12/Driver/Reference Generator ==
  Driver_Information : Inport
  steering_angle : Inport  Port=2
  Bus Creator : BusCreator  Inputs=Reference,Driver
  Bus Creator1 : BusCreator  Inputs=9
  Bus Selector2 : BusSelector  OutputSignals=Driver.y,Driver.x,Reference.y_ref,Reference.x_ref  OutputAsBus=on
  Memory : Memory  InitialCondition=1
  Mutiple XY Graph : Subsystem  mask(Mutiple XY Graph){number_of_trajectories=2, axis_limits=[-100 10 -25 90], sample_time=0.15}
      mask prompts: number_of_trajectories "Number of Trajectories"; axis_limits "Axis Limits"; sample_time "Sample Time"
      mask Display: plot([.05 .95 .95 .05 .05],[.45 .45 .95 .95 .45], 0.5+cos(0:0.1:2*pi)*0.3,0.7+sin(0:0.1:2*pi)*0.2)
  Reference Geneator : MATLAB Function  TreatAsAtomicUnit=on  SystemSampleTime=t
  Selector : BusSelector  OutputSignals=psi,Vg,yaw,x,y
  Subsystem : Subsystem
  Unit Delay : UnitDelay  SampleTime=-1  HasFrameUpgradeWarning=on
  Unit Delay2 : UnitDelay  SampleTime=-1  HasFrameUpgradeWarning=on
  Vg_ref : Constant  Value=8
  Controller Information : Outport
  wires:
  Vg_ref/1 -> Reference Geneator/3(Vg_ref)
  Driver_Information/1 -> Bus Creator/2, Selector/1  "Driver"
  Selector/1 -> Subsystem/1(<psi>)  "<psi>"
  Reference Geneator/3(d_error) -> Bus Creator1/2
  Bus Creator1/1 -> Bus Creator/1  "Reference"
  Bus Selector2/1 -> Mutiple XY Graph/1(In1)
  Selector/2 -> Reference Geneator/5(Vg)  "<Vg>"
  Reference Geneator/2(v_error) -> Bus Creator1/1
  Reference Geneator/5(v_cog) -> Bus Creator1/4  "v_cog"
  Selector/3 -> Reference Geneator/6(yaw)  "<yaw>"
  Bus Creator/1 -> Controller Information/1, Bus Selector2/1
  Selector/5 -> Reference Geneator/8(y)  "<y>"
  Selector/4 -> Reference Geneator/7(x)  "<x>"
  Subsystem/1(psi_rev) -> Reference Geneator/4(psi)
  Reference Geneator/4(psi_error) -> Bus Creator1/3
  Reference Geneator/1(index) -> Memory/1
  Memory/1 -> Reference Geneator/1("index ")
  Reference Geneator/6(r_ref) -> Bus Creator1/5
  Reference Geneator/7(r_error_2) -> Bus Creator1/6
  steering_angle/1 -> Reference Geneator/2(steering_angle)  "Driver"
  Reference Geneator/11(counter) -> Unit Delay/1
  Unit Delay/1 -> Reference Geneator/10("counter ")
  Reference Geneator/10(wind_down) -> Bus Creator1/9, Unit Delay2/1
  Unit Delay2/1 -> Reference Geneator/9("wind_down ")
  Reference Geneator/8(x_ref) -> Bus Creator1/7
  Reference Geneator/9(y_ref) -> Bus Creator1/8

== system complete_plant_ediff_conflict_copy_Ethan’s MacBook Pro_2022_11_12/Vehicle Model/Powertrain ==
  TV Torque : Inport
  Motor Shaft Angular Speed : Inport  Port=2
  Gearbox : Subsystem
  Motor and Battery : Subsystem
      settings: PortSchema="{\"entries\":[{\"content\":{\"sides\":[{\"content\":{\"connectorIds\":[\"Out1\",\"Out2\",\"Out3\"]},\"type\":\"ConnectorPlacement.EquallySpacedRectSide\",\"uuid\":\"0a1f914b-70eb-46fa-9e3d-552685e5145b\"},{\"content\":{\"connectorIds\":[\"In1\",\"In2\"],\"side\":\"RIGHT\"},\"type\":\"ConnectorPlacement.EquallySpacedRectSide\",\"uuid\":\"3f4913ad-53b1-4c2d-9942-63851d66d84d\"},{\"content\":{\"connectorIds\":[],\"side\":\"TOP\"},\"type\":\"ConnectorPlacement.EquallySpacedRectSide\",\"uuid\":\"355326fa-9c02-45e7-a319-d2a0d6b3d4bd\"},{\"content\":{\"connectorIds\":[],\"side\":\"HIDDEN\"},\"type\":\"ConnectorPlacement.EquallySpacedRectSide\",\"uuid\":\"65af7ff0-f0aa-4be0-a188-dc3dcb8956e6\"}]},\"type\":\"ConnectorPlacement.EquallySpacedConnector\",\"uuid\":\"023a46d9-a637-4c8e-84c1-6893dcef87c2\"}],\"packageUris\":[\"http://schema.mathworks.com/mf0/Connector/R2020b\"],\"version\":\"1.0\"}"
  power_limits : Outport
  Battery Voltage : Outport  Port=2
  AxlTrq : Outport  Port=3
  wires:
  TV Torque/1 -> Motor and Battery/2(TV Torque)
  Motor and Battery/1(Motor Torque) -> Gearbox/1(Sun Gear Torque)
  Motor and Battery/2(power_limits) -> power_limits/1
  Motor Shaft Angular Speed/1 -> Motor and Battery/1(Motor Shaft Angular Speed)
  Gearbox/1(AxlTrq) -> AxlTrq/1
  Motor and Battery/3(Battery Voltage) -> Battery Voltage/1

== system complete_plant_ediff_conflict_copy_Ethan’s MacBook Pro_2022_11_12/Vehicle Model/Suspension ==
  Steering : Inport
  Vehicle : Inport  Port=2
  Wheel : Inport  Port=3
  Double Wishbone Suspension : Subsystem  VariantControl=1
      mask Display: image('suspdw.png');
  Independent Mapped Front Suspension Mapped Solid Axle Rear Suspension : Subsystem  VariantControl=2
      mask Display: image([imread('suspindmap.png');imread('suspsamap.png')]);
  Kinematics and Compliance Independent Suspension : Subsystem  VariantControl=6
      mask Display: image('suspkandc.png');
  MacPherson Front Suspension Solid Axle Rear Suspension : Subsystem  VariantControl=3
      mask Display: image([imread('suspmacp.png');imread('suspsacoil.png')]);
  MacPherson Suspension : Subsystem  VariantControl=4
      mask Display: image('suspmacp.png');
  Mapped Suspension : Subsystem  VariantControl=5
      mask Display: image('suspindmap.png');
  Suspension : Outport  VectorParamsAs1DForOutWhenUnconnected=off

== system complete_plant_ediff_conflict_copy_Ethan’s MacBook Pro_2022_11_12/Vehicle Model/Vehicle ==
  Suspension : Inport
  Wind : Inport  Port=2
  Variant Subsystem : Subsystem  Variant=on  VariantControlMode=label  LabelModeActiveChoice=1
  VehFdbk : Outport  VectorParamsAs1DForOutWhenUnconnected=off
  wires:
  Variant Subsystem/1(VehFdbk) -> VehFdbk/1  "VehFdbk"
  Wind/1 -> Variant Subsystem/2(Wind)
  Suspension/1 -> Variant Subsystem/1(Suspension)

== system complete_plant_ediff_conflict_copy_Ethan’s MacBook Pro_2022_11_12/Vehicle Model/Visualization1 ==
  VehFdbk : Inport
  Wheels : Inport  Port=2
  Bus Selector1 : BusSelector  OutputSignals=InertFrm.Cg.Ang.phi,InertFrm.Cg.Ang.theta,InertFrm.Cg.Ang.psi  OutputAsBus=on
  Bus Selector10 : BusSelector  OutputSignals=BdyFrm.Forces.FrntAxl.Lft.Fy,BdyFrm.Forces.FrntAxl.Rght.Fy,BdyFrm.Forces.RearAxl.Lft.Fy,BdyFrm.Forces.RearAxl.Rght.Fy
  Bus Selector2 : BusSelector  OutputSignals=BdyFrm.Forces.FrntAxl.Lft.Fx,BdyFrm.Forces.FrntAxl.Rght.Fx,BdyFrm.Forces.RearAxl.Lft.Fx,BdyFrm.Forces.RearAxl.Rght.Fx
  Bus Selector5 : BusSelector  OutputSignals=Steering.WhlAng  OutputAsBus=on
  Bus Selector6 : BusSelector  OutputSignals=InertFrm.Cg.Disp.X,InertFrm.Cg.Disp.Y,InertFrm.Cg.Disp.Z  OutputAsBus=on
  Bus Selector7 : BusSelector  OutputSignals=InertFrm.Cg.Vel.Xdot,InertFrm.Cg.Vel.Ydot,InertFrm.Cg.Vel.Zdot  OutputAsBus=on
  Bus to Vector{,1..3} (4 alike) : BusToVector
  Ground1 : Ground
  Mux : Mux  Inputs=3
  Mux1 : Mux
  Mux2 : Mux
  Vehicle XY Plotter : vehdynlibviscommon/Vehicle XY Plot Configuration  extRef=on  extStats=off  extTireF=on  a=0.7922471  b=0.7828529  w=1.26  figBorder=10  bufferSize=1024  velNorm=5  tireFNorm=1000  pltDT=.1
  wires:
  Bus Selector1/1 -> Bus to Vector2/1
  VehFdbk/1 -> Bus Selector10/1, Bus Selector2/1, Bus Selector6/1, Bus Selector1/1, Bus Selector7/1
  Mux/1 -> Vehicle XY Plotter/5
  Bus Selector7/1 -> Bus to Vector1/1
  Bus to Vector2/1 -> Vehicle XY Plotter/2
  Bus to Vector1/1 -> Vehicle XY Plotter/3
  Bus Selector6/1 -> Bus to Vector/1
  Bus to Vector/1 -> Vehicle XY Plotter/1
  Ground1/1 -> Mux/3, Mux/2, Mux/1
  Bus to Vector3/1 -> Vehicle XY Plotter/4
  Bus Selector5/1 -> Bus to Vector3/1
  Wheels/1 -> Bus Selector5/1
  Mux1/1 -> Vehicle XY Plotter/6
  Bus Selector2/1 -> Mux1/1  "<Fx>"
  Bus Selector2/2 -> Mux1/2  "<Fx>"
  Bus Selector2/3 -> Mux1/3  "<Fx>"
  Bus Selector2/4 -> Mux1/4  "<Fx>"
  Mux2/1 -> Vehicle XY Plotter/7
  Bus Selector10/1 -> Mux2/1  "<Fy>"
  Bus Selector10/2 -> Mux2/2  "<Fy>"
  Bus Selector10/3 -> Mux2/3  "<Fy>"
  Bus Selector10/4 -> Mux2/4  "<Fy>"

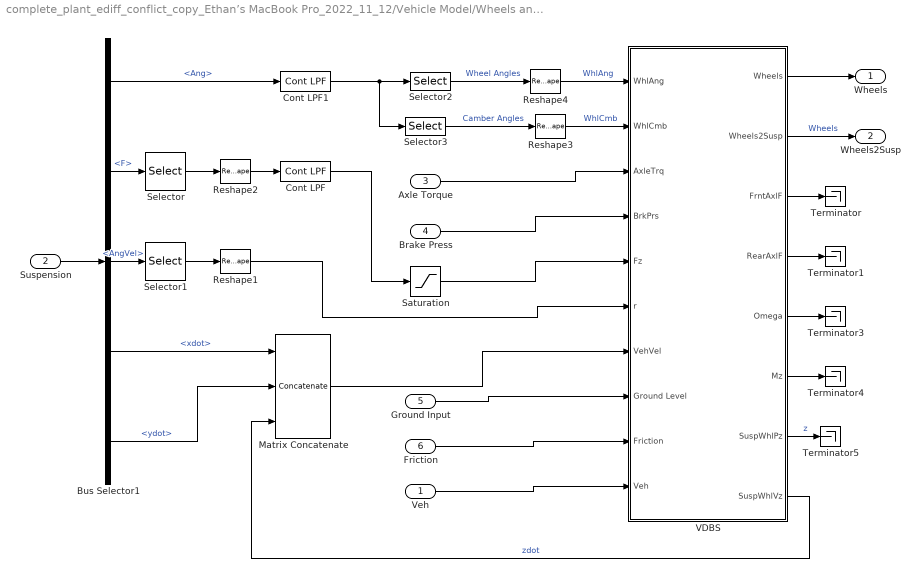
== system complete_plant_ediff_conflict_copy_Ethan’s MacBook Pro_2022_11_12/Vehicle Model/Wheels and Tires ==
  Veh : Inport
  Suspension : Inport  Port=2
  Axle Torque : Inport  Port=3
  Brake Press : Inport  Port=4  Unit=Pa
  Ground Input : Inport  Port=5
  Friction : Inport  Port=6  PortDimensions=4
  Bus Selector1 : BusSelector  OutputSignals=Whl.Ang,Whl.F,Whl.AngVel,Whl.xdot,Whl.ydot
  Cont LPF : autolibutils/Cont LPF  wc=100*2*pi  AbsoluteTolerance=auto  aMode=2
  Cont LPF1 : autolibutils/Cont LPF  wc=100*2*pi  AbsoluteTolerance=auto  aMode=2
  Matrix Concatenate : Concatenate  NumInputs=3  Mode=Multidimensional array
  Reshape{1..4} (4 alike) : Reshape
  Saturation : Saturate  UpperLimit=inf  LowerLimit=-10*9.81*2000  ZeroCross=off
  Selector : Selector  NumberOfDimensions=2  InputPortWidth=3  IndexOptions=Index vector (dialog),Select all  Indices=[3],1  OutputSizes=1,1
  Selector1 : Selector  NumberOfDimensions=2  InputPortWidth=1  IndexOptions=Index vector (dialog),Select all  Indices=[3],1  OutputSizes=1,1
  Selector2 : Selector  NumberOfDimensions=2  InputPortWidth=3  IndexOptions=Index vector (dialog),Select all  Indices=3,1  OutputSizes=1,1
  Selector3 : Selector  NumberOfDimensions=2  InputPortWidth=3  IndexOptions=Index vector (dialog),Select all  Indices=1,1  OutputSizes=1,1
  Terminator{,1,3..5} (5 alike) : Terminator
  VDBS : Subsystem  VariantControl=0
  Wheels : Outport  VectorParamsAs1DForOutWhenUnconnected=off
  Wheels2Susp : Outport  Port=2  VectorParamsAs1DForOutWhenUnconnected=off
  wires:
  Bus Selector1/2 -> Selector/1  "<F>"
  VDBS/3(FrntAxlF) -> Terminator/1
  VDBS/4(RearAxlF) -> Terminator1/1
  VDBS/5(Omega) -> Terminator3/1
  VDBS/6(Mz) -> Terminator4/1
  Selector1/1 -> Reshape1/1
  Matrix Concatenate/1 -> VDBS/7(VehVel)
  Axle Torque/1 -> VDBS/3(AxleTrq)
  Reshape4/1 -> VDBS/1(WhlAng)  "WhlAng"
  Reshape3/1 -> VDBS/2(WhlCmb)  "WhlCmb"
  Selector/1 -> Reshape2/1
  Saturation/1 -> VDBS/5(Fz)
  Ground Input/1 -> VDBS/8(Ground Level)
  VDBS/8(SuspWhlVz) -> Matrix Concatenate/3  "zdot"
  Bus Selector1/1 -> Cont LPF1/1  "<Ang>"
  Selector3/1 -> Reshape3/1  "Camber Angles"
  Suspension/1 -> Bus Selector1/1
  Bus Selector1/4 -> Matrix Concatenate/1  "<xdot>"
  Bus Selector1/5 -> Matrix Concatenate/2  "<ydot>"
  VDBS/7(SuspWhlPz) -> Terminator5/1  "z"
  Reshape2/1 -> Cont LPF/1
  Bus Selector1/3 -> Selector1/1  "<AngVel>"
  Reshape1/1 -> VDBS/6(r)
  Brake Press/1 -> VDBS/4(BrkPrs)
  Friction/1 -> VDBS/9(Friction)
  Cont LPF/1 -> Saturation/1
  Cont LPF1/1 -> Selector3/1, Selector2/1
  Selector2/1 -> Reshape4/1  "Wheel Angles"
  Veh/1 -> VDBS/10(Veh)
  VDBS/2(Wheels2Susp) -> Wheels2Susp/1  "Wheels"
  VDBS/1(Wheels) -> Wheels/1

== system complete_plant_ediff_conflict_copy_Ethan’s MacBook Pro_2022_11_12/Driver/Lateral Control/Lateral Controller ==
  r_error : Inport
  d_error : Inport  Port=2
  <Vg> : Inport  Port=3
  angle_error : Inport  Port=4
  wind_down : Inport  Port=5
  Add Constant : Bias  Bias=0.1  SaturateOnIntegerOverflow=off
  Discrete-Time Integrator : DiscreteIntegrator  IntegratorMethod=Accumulation: Backward Euler  gainval=30  ExternalReset=level  SampleTime=-1  LimitOutput=on  UpperSaturationLimit=110  LowerSaturationLimit=-110  ICPrevOutput=DiscIntNeverNeededParam  ICPrevScaledInput=DiscIntNeverNeededParam
  Divide : Product  Inputs=*/
  Gain3 : Gain  Gain=2
  Gain4 : Gain  Gain=0
  IC : InitialCondition  Value=0
  PID Controller : slpidlib/PID Controller  Controller=PID  Form=Parallel  TimeDomain=Discrete-time  UseExternalTs=off  SampleTime=-1  IntegratorMethod=Forward Euler  FilterMethod=Forward Euler  ControllerParametersSource=internal  P=100  I=0  UseKiTs=off  D=0  N=0  UseFilter=on  TunerSelectOption=Transfer Function Based (PID Tuner App)  InitialConditionSource=internal  InitialConditionForIntegrator=0  InitialConditionForFilter=0  DifferentiatorICPrevScaledInput=0  ExternalReset=none  TrackingMode=off  Kt=1  LimitOutput=on  SatLimitsSource=internal  UpperSaturationLimit=40  LowerSaturationLimit=-40  LinearizeAsGain=on  AntiWindupMode=none  Kb=1  LimitIntegrator=off  UpperIntegratorSaturationLimit=inf  LowerIntegratorSaturationLimit=-inf  POutMin=[]  POutMax=[]  IOutMin=[]  IOutMax=[]  DOutMin=[]  DOutMax=[]  NOutMin=[]  NOutMax=[]  SumOutMin=[]  SumOutMax=[]  SaturationOutMin=[]  SaturationOutMax=[]  PParamMin=[]  PParamMax=[]  IParamMin=[]  IParamMax=[]  DParamMin=[]  DParamMax=[]  NParamMin=[]  NParamMax=[]  KbParamMin=[]  KbParamMax=[]  KtParamMin=[]  KtParamMax=[]  KbOutMin=[]  KbOutMax=[]  KtOutMin=[]  KtOutMax=[]  IntegratorOutMin=[]  IntegratorOutMax=[]  FilterOutMin=[]  FilterOutMax=[]  SumI1OutMin=[]  SumI1OutMax=[]  SumI2OutMin=[]  SumI2OutMax=[]  SumI3OutMin=[]  SumI3OutMax=[]  SumI4OutMin=[]  SumI4OutMax=[]  SumDOutMin=[]  SumDOutMax=[]  DifferentiatorOutMin=[]  DifferentiatorOutMax=[]  FilterDiffOutCoefMin=[]  FilterDiffOutCoefMax=[]  ReciprocalOutMin=[]  ReciprocalOutMax=[]  SumDenOutMin=[]  SumDenOutMax=[]  SumNumOutMin=[]  SumNumOutMax=[]  DivideOutMin=[]  DivideOutMax=[]  UdiffTsProdOutMin=[]  UdiffTsProdOutMax=[]  NTsProdOutMin=[]  NTsProdOutMax=[]  UintegralTsProdOutMin=[]  UintegralTsProdOutMax=[]  UngainTsProdOutMin=[]  UngainTsProdOutMax=[]  ClampingZeroOutDataTypeStr=Inherit: Inherit via back propagation  ClampingZeroOutMin=[]  ClampingZeroOutMax=[]  FilterDenConstantOutDataTypeStr=Inherit: Inherit via back propagation  FilterDenConstantOutMin=[]  FilterDenConstantOutMax=[]  PCopyOutDataTypeStr=Inherit: Inherit via back propagation  PCopyOutMin=[]  PCopyOutMax=[]  NCopyOutDataTypeStr=Inherit: Inherit via back propagation  NCopyOutMin=[]  NCopyOutMax=[]  IntegratorContinuousStateAttributes=''  IntegratorStateMustResolveToSignalObject=off  IntegratorRTWStateStorageClass=Auto  FilterContinuousStateAttributes=''  FilterStateMustResolveToSignalObject=off  FilterRTWStateStorageClass=Auto  ParallelPVariant=InternalParameters  IdealPVariant=Disabled  IVariant=InternalParameters  DVariant=InternalParameters  IntegratorVariant=Discrete  SatVariant=Enabled  AWVariant=Passthrough  PCopyVariant=Disabled  TRVariant=Disabled  FdbkBlocksVariant=Forward  IdealPFdbkVariant=Disabled  SatFdbkVariant=Disabled  DerivativeFilterVariant=ForwardEulerFilter  NVariant=InternalParameters  NCopyVariant=Disabled  FilterICVariant=InternalICsFilter  IntegratorICVariant=InternalICs  ExternalResetVariant=Disabled  TRSumVariant=Passthrough  SumFdbkVariant=Disabled  SumVariant=Sum_PID  TsampFilterVariant=InternalTs  TsampNgainVariant=Passthrough  TsampIntegralVariant=Passthrough  ExternalSaturationOutDataTypeStr=Inherit: Same as second input
  PID Controller1 : slpidlib/PID Controller  Controller=PID  Form=Parallel  TimeDomain=Discrete-time  UseExternalTs=off  SampleTime=-1  IntegratorMethod=Forward Euler  FilterMethod=Forward Euler  ControllerParametersSource=internal  P=1  I=0  UseKiTs=off  D=0.3  N=45  UseFilter=on  TunerSelectOption=Transfer Function Based (PID Tuner App)  InitialConditionSource=internal  InitialConditionForIntegrator=0  InitialConditionForFilter=0  DifferentiatorICPrevScaledInput=0  ExternalReset=none  TrackingMode=off  Kt=1  LimitOutput=on  SatLimitsSource=internal  UpperSaturationLimit=40  LowerSaturationLimit=-40  LinearizeAsGain=on  AntiWindupMode=none  Kb=1  LimitIntegrator=off  UpperIntegratorSaturationLimit=inf  LowerIntegratorSaturationLimit=-inf  POutMin=[]  POutMax=[]  IOutMin=[]  IOutMax=[]  DOutMin=[]  DOutMax=[]  NOutMin=[]  NOutMax=[]  SumOutMin=[]  SumOutMax=[]  SaturationOutMin=[]  SaturationOutMax=[]  PParamMin=[]  PParamMax=[]  IParamMin=[]  IParamMax=[]  DParamMin=[]  DParamMax=[]  NParamMin=[]  NParamMax=[]  KbParamMin=[]  KbParamMax=[]  KtParamMin=[]  KtParamMax=[]  KbOutMin=[]  KbOutMax=[]  KtOutMin=[]  KtOutMax=[]  IntegratorOutMin=[]  IntegratorOutMax=[]  FilterOutMin=[]  FilterOutMax=[]  SumI1OutMin=[]  SumI1OutMax=[]  SumI2OutMin=[]  SumI2OutMax=[]  SumI3OutMin=[]  SumI3OutMax=[]  SumI4OutMin=[]  SumI4OutMax=[]  SumDOutMin=[]  SumDOutMax=[]  DifferentiatorOutMin=[]  DifferentiatorOutMax=[]  FilterDiffOutCoefMin=[]  FilterDiffOutCoefMax=[]  ReciprocalOutMin=[]  ReciprocalOutMax=[]  SumDenOutMin=[]  SumDenOutMax=[]  SumNumOutMin=[]  SumNumOutMax=[]  DivideOutMin=[]  DivideOutMax=[]  UdiffTsProdOutMin=[]  UdiffTsProdOutMax=[]  NTsProdOutMin=[]  NTsProdOutMax=[]  UintegralTsProdOutMin=[]  UintegralTsProdOutMax=[]  UngainTsProdOutMin=[]  UngainTsProdOutMax=[]  ClampingZeroOutDataTypeStr=Inherit: Inherit via back propagation  ClampingZeroOutMin=[]  ClampingZeroOutMax=[]  FilterDenConstantOutDataTypeStr=Inherit: Inherit via back propagation  FilterDenConstantOutMin=[]  FilterDenConstantOutMax=[]  PCopyOutDataTypeStr=Inherit: Inherit via back propagation  PCopyOutMin=[]  PCopyOutMax=[]  NCopyOutDataTypeStr=Inherit: Inherit via back propagation  NCopyOutMin=[]  NCopyOutMax=[]  IntegratorContinuousStateAttributes=''  IntegratorStateMustResolveToSignalObject=off  IntegratorRTWStateStorageClass=Auto  FilterContinuousStateAttributes=''  FilterStateMustResolveToSignalObject=off  FilterRTWStateStorageClass=Auto  ParallelPVariant=InternalParameters  IdealPVariant=Disabled  IVariant=InternalParameters  DVariant=InternalParameters  IntegratorVariant=Discrete  SatVariant=Enabled  AWVariant=Passthrough  PCopyVariant=Disabled  TRVariant=Disabled  FdbkBlocksVariant=Forward  IdealPFdbkVariant=Disabled  SatFdbkVariant=Disabled  DerivativeFilterVariant=ForwardEulerFilter  NVariant=InternalParameters  NCopyVariant=Disabled  FilterICVariant=InternalICsFilter  IntegratorICVariant=InternalICs  ExternalResetVariant=Disabled  TRSumVariant=Passthrough  SumFdbkVariant=Disabled  SumVariant=Sum_PID  TsampFilterVariant=InternalTs  TsampNgainVariant=Passthrough  TsampIntegralVariant=Passthrough  ExternalSaturationOutDataTypeStr=Inherit: Same as second input
  Rate Limiter : RateLimiter  RisingSlewLimit=360  FallingSlewLimit=-360  SampleTimeMode=inherited
  Saturation : Saturate  UpperLimit=100  LowerLimit=-100
  Saturation1 : Saturate  UpperLimit=45  LowerLimit=-45
  Saturation2 : Saturate  UpperLimit=130  LowerLimit=-130
  Saturation3 : Saturate  UpperLimit=130  LowerLimit=-130
  Subsystem : Subsystem
      settings: PortSchema="{\"entries\":[{\"content\":{\"sides\":[{\"content\":{\"connectorIds\":[\"In1\",\"In2\",\"In3\"]},\"type\":\"ConnectorPlacement.EquallySpacedRectSide\",\"uuid\":\"a45e5e90-b109-401e-aae9-d94d2084e52d\"},{\"content\":{\"connectorIds\":[\"In4\",\"Out1\",\"Out2\"],\"side\":\"RIGHT\"},\"type\":\"ConnectorPlacement.EquallySpacedRectSide\",\"uuid\":\"6672bef5-f603-4fc1-bd56-f951bac9a521\"},{\"content\":{\"connectorIds\":[],\"side\":\"TOP\"},\"type\":\"ConnectorPlacement.EquallySpacedRectSide\",\"uuid\":\"eb691037-3ca8-41fa-a87f-0e9f75ad26f8\"}]},\"type\":\"ConnectorPlacement.EquallySpacedConnector\",\"uuid\":\"41304219-e0b3-4eff-bc9b-9bcf52681ed9\"}],\"packageUris\":[\"http://schema.mathworks.com/mf0/Connector/R2020b\"],\"version\":\"1.0\"}"
  Sum : Sum  Inputs=+++
  Sum4 : Sum  Inputs=|++
  steering_angle : Outport
  wires:
  <Vg>/1 -> Add Constant/1
  Add Constant/1 -> Divide/2
  PID Controller/1 -> Sum/2
  Gain3/1 -> Gain4/1, Subsystem/1(In2)
  d_error/1 -> Divide/1
  Saturation/1 -> Sum4/1
  Gain4/1 -> Saturation/1
  Saturation1/1 -> Sum/3
  PID Controller1/1 -> Saturation1/1
  IC/1 -> Gain3/1, Subsystem/2(In1)
  Divide/1 -> PID Controller/1
  Sum4/1 -> Saturation3/1
  Saturation3/1 -> Sum/1
  Discrete-Time Integrator/1 -> Sum4/2, Subsystem/4(In3)
  angle_error/1 -> PID Controller1/1
  wind_down/1 -> Subsystem/3(In4)
  Subsystem/1(Out1) -> Discrete-Time Integrator/1
  Subsystem/2(Out2) -> Discrete-Time Integrator/2
  Sum/1 -> Rate Limiter/1
  Rate Limiter/1 -> Saturation2/1
  Saturation2/1 -> steering_angle/1
  r_error/1 -> IC/1

== system complete_plant_ediff_conflict_copy_Ethan’s MacBook Pro_2022_11_12/Driver/Reference Generator/Mutiple XY Graph ==
  In1 : Inport
  Level-2 MATLAB S-Function : M-S-Function  FunctionName=multiple_xy_graph  Parameters=number_of_trajectories,axis_limits
  Rate Transition : RateTransition  OutPortSampleTime=sample_time
  wires:
  In1/1 -> Rate Transition/1
  Rate Transition/1 -> Level-2 MATLAB S-Function/1

== system complete_plant_ediff_conflict_copy_Ethan’s MacBook Pro_2022_11_12/Driver/Reference Generator/Subsystem ==
  <psi> : Inport  PortDimensions=1
  Constant1 : Constant  Value=2*pi
  Constant2 : Constant  Value=pi
  Constant3 : Constant  Value=-pi
  Constant4 : Constant  Value=2*pi
  Constant5 : Constant  Value=-2*pi
  GreaterThan : RelationalOperator  Operator=>  OutDataTypeStr=boolean  RndMeth=Simplest  InputSameDT=off
  Less Than : RelationalOperator  Operator=<  OutDataTypeStr=boolean  RndMeth=Simplest  InputSameDT=off
  Mod : Math  Operator=mod
  Product : Product
  Product1 : Product
  Sum : Sum  Inputs=+++
  psi_rev : Outport
  wires:
  Product1/1 -> Sum/3
  Less Than/1 -> Product1/2
  GreaterThan/1 -> Product/1
  Mod/1 -> GreaterThan/1, Sum/1, Less Than/1
  Constant1/1 -> Mod/2
  Constant5/1 -> Product/2
  Constant3/1 -> Less Than/2
  Constant4/1 -> Product1/1
  Constant2/1 -> GreaterThan/2
  Product/1 -> Sum/2
  <psi>/1 -> Mod/1
  Sum/1 -> psi_rev/1
